simulink model "stream_output_window_input"  (R2019b)
settings: Solver=VariableStepAuto  StartTime=0.0  StopTime=128  RelTol=1e-3
undefined symbols (not defined in the file): xc7vx485tffg1157
libraries: ModelComposer x5
settings Model: Creator=viswanad  LastModifiedBy=abehbood
settings DataIOCC: ReturnWorkspaceOutputs=off
settings SFSimCC: CustomCodeUndefinedFunction=UseInterfaceOnly

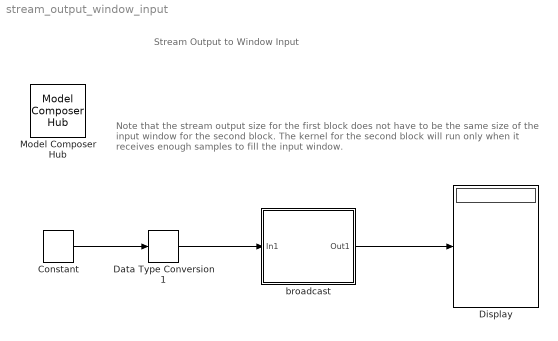
== system stream_output_window_input ==
  note: Stream Output to Window Input
  note: Note that the stream output size for the first block does not have to be the
      | same size of the input window for the second block. The kernel for the second block will
      | run only when it receives enough samples to fill the input window.
  Constant : ModelComposer/Constant  Value=[1 2 3 4 5 6 7 8]  SampleTime=1  OutDataType=double  TypeExp=''  Signedness=Signed  WordLength=16  FractionalLength=0  RoundingMode=Truncation to minus infinity  OverflowMode=Wrap around
  Data Type Conversion1 : ModelComposer/Data Type Conversion  OutDataType=int32  TypeExp=''  Signedness=Signed  WordLength=16  FractionalLength=0  RoundingMode=Truncation to minus infinity  OverflowMode=Wrap around
  Display : Display
  Model Composer Hub : ModelComposer/Model Composer Hub  CodeGeneration=off  SubsystemName=broadcast  TargetDirectory=./code9_template_template  ExportType=AI Engines  IpVendor=xilinx.com  IpLibrary=hls  IpVersion=1.0  IpHWLanguage=Verilog  AieCompilerOptions={}  CreateTestbench=on  TestbenchStackSize=10  RunAieSim=on  AieSimTimeout=50000  LaunchVitisAnalyzer=off  RunX86Sim=off  X86SimTimeout=10  ProjDevice=xc7vx485tffg1157-1  ProjDevicePart=xc7vx485tffg1157-1  SamplePeriod=-1  ClockFrequency=200  DataPathParallelism=1
  broadcast : Subsystem
  wires:
  Constant/1 -> Data Type Conversion1/1
  broadcast/1(Out1) -> Display/1
  Data Type Conversion1/1 -> broadcast/1(In1)

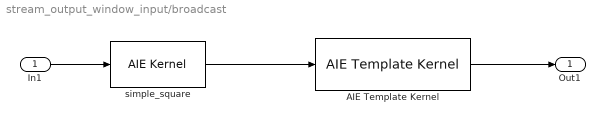
== system stream_output_window_input/broadcast ==
  In1 : Inport
  AIE Template Kernel : ModelComposer/AIE Template Kernel  KernelAllAttrs=s[12;12;9;9;19;14;21;23;24;21;12;24;26;26;26;27;28;9;21;23;23;23;24;25;14;19;19;29]@FunctionNameDeclFileNamePortNamesPortTypesPortSerializedTypesPortDirectionsPortWindowSizeEnablesPortWindowMarginEnablesPortSynchronicityEnablesPortSignalSizeEnablesFunctionDeclFunctionTemplateSpecKindFunctionTemplateParamNamesFunctionTemplateParamKindsFunctionTemplateParamTypesFunctionTemplateParamValuesFunctionTemplateParamEnablesClassDeclClassTemplateSpecKindClassTemplateParamNamesClassTemplateParamKindsClassTemplateParamTypesClassTemplateParamValuesClassTemplateParamEnablesClassCtorDeclsClassCtorParamNamesClassCtorParamTypesClassCtorParamSerializedTypes[1 1]@C[28 1]@t19@pass_through_kernelt49@../../src/kernels/window_in_window_out_template.hC[2 1]@t3@inwt4@outwC[2 1]@t20@input_window_int32 *t21@output_window_int32 *C[2 1]@t30@{P{Tinput_window{1{t{Bi32}}}}}t31@{P{Toutput_window{1{t{Bi32}}}}}C[2 1]@t5@inputt6@outputC[2 1]@l1@l1@C[2 1]@l1@l0@C[2 1]@l1@l1@C[2 1]@l0@l0@t107@template < int NUM_SAMPLES > void pass_through_kernel(input_window_int32 * inw, output_window_int32 * outw)t8@implicitC[1 1]@t11@NUM_SAMPLESC[1 1]@t7@nontypeC[1 1]@t3@intC[1 1]@nC[1 1]@l1@nne[0 1]@e[0 1]@e[0 1]@e[0 1]@e[0 1]@e[0 1]@e[0 1]@e[0 1]@e[0 1]@  PortNames={'inw'; 'outw'}  PortSerializedTypes={'{P{Tinput_window{1{t{Bi32}}}}}'; '{P{Toutput_window{1{t{Bi32}}}}}'}  PortWindowSizes={1.600000000000000000e+01; 1.600000000000000000e+01}  PortWindowMargins={0.000000000000000000e+00; 0.000000000000000000e+00}  PortSynchronicities={'auto'; 'auto'}  PortSignalSizes={0.000000000000000000e+00; 0.000000000000000000e+00}  FunctionTemplateSpecKind=implicit  FunctionTemplateParamNames={'NUM_SAMPLES'}  FunctionTemplateParamKinds={'nontype'}  FunctionTemplateParamTypes={'int'}  FunctionTemplateParamValues={'0'}  FunctionIndex=1  FunctionTabVisible=on  FunctionTemplateParamsVisible=on  FunctionDeclTypeOptions=C[1 1]@t107@template < int NUM_SAMPLES > void pass_through_kernel(input_window_int32 * inw, output_window_int32 * outw)  FunctionDecl=template < int NUM_SAMPLES > void pass_through_kernel(input_window_int32 * inw, output_window_int32 * outw)  FunctionTemplateParams={ 'NUM_SAMPLES', 'int', '' }  FunctionTemplateParamsEnables={'off', 'off', 'on'}  PortAttrs={ 'input', 'inw', 'input_window_int32 *', '16', '0', 'auto', ''; 'output', 'outw', 'output_window_int32 *', '16', '', 'auto', '' }  PortAttrsEnables={'off', 'off', 'off', 'on', 'on', 'on', 'off';'off', 'off', 'off', 'on', 'off', 'on', 'off'}  KernelHeaderFile=src/kernels/window_in_window_out_template.h  KernelFunction=pass_through_kernel  KernelSourceFile=src/kernels/window_in_window_out_template.cc  KernelSearchPaths={}  PreProcOptions={}  CoreRuntimeRatio=0.9  KernelLocSpec=off  ColRowLocation=[0 0]
  simple_square : ModelComposer/AIE Kernel  PortAttributesTable={ 'Input', 'in', 'input_stream_int32 *', '', '', '', ''; 'Output', 'out', 'output_stream_int32 *', '', '', '', '8' }  PortAttributesEnablement={'off', 'off', 'off', 'off', 'off', 'off', 'off';'off', 'off', 'off', 'off', 'off', 'off', 'on'}  FormalArgDecls={'input_stream_int32 * in', 'output_stream_int32 * out'}  PortWindowSizes={0.000000000000000000e+00; 0.000000000000000000e+00}  PortWindowMargins={0.000000000000000000e+00; 0.000000000000000000e+00}  PortSynchronicities={'auto'; 'auto'}  PortSignalSizes={0.000000000000000000e+00; 8.000000000000000000e+00}  SimLibPath=''  FunctionTabVisible=on  FunctionDescription=void simple_square(input_stream_int32 * in, output_stream_int32 * out)  KernelHeaderFile=src/kernels/stream_in_stream_out.h  KernelFunction=simple_square  KernelFunctionSelect=<empty>  KernelSourceFile=src/kernels/stream_in_stream_out.cc  KernelSearchPaths={}  PreProcOptions={}  CoreRuntimeRatio=0.9  KernelLocSpec=off  ColRowLocation=[0 0]
  Out1 : Outport
  wires:
  In1/1 -> simple_square/1
  AIE Template Kernel/1 -> Out1/1
  simple_square/1 -> AIE Template Kernel/1
